simulink model "sldemo_hydcyl"  (Simulink 7.6)
settings: Solver=ode45  SolverMode=SingleTasking  StartTime=0  StopTime=0.1  RelTol=1e-4  AbsTol=1e-6
model workspace (MATLAB code in the model file):
  | % Load the initial conditions and initialization data
  | % Using the same MAT file as
  | % sldemo_hydcyl.mdl
  | % sldemo_hydcyl4.mdl
  | % sldemo_hydrod.mdl
  | 
  | load sldemo_hydcyl_data;
undefined symbols (not defined in the file or in its folder): C2, K, Qmax
libraries: hydlib x2
Description:
  | Single Hydraulic Cylinder Simulation
  | 
  | This demo uses Simulink(R) to model a hydraulic cylinder. You can apply these
  | concepts to applications where you need to model hydraulic behavior. See two
  | related demos that use the same basic components:
  | 
  | * four cylinder model: sldemo_hydcyl4.mdl
  | * two cylinder model with load constraints: sldemo_hydrod.mdl
settings Model: Creator=The MathWorks Inc.  CovMetricSettings=d  ExtModeTrigMode=oneshot  ExtModeArmWhenConnect=off  ExtModeAutoUpdateStatusClock=off  BufferReuse=off
settings DataIOCC: LimitDataPoints=off  SaveOutput=off  SaveTime=off  SignalLoggingName=sldemo_hydcyl_output
settings OptimizationCC: BlockReduction=off  BooleanDataType=off  ConditionallyExecuteInputs=off  InlineInvariantSignals=on  OptimizeBlockIOStorage=off  BufferReuse=off  ExpressionFolding=off  LocalBlockOutputs=off  InitFltsAndDblsToZero=on  BufferReusableBoundary=off
settings DebuggingCC: AlgebraicLoopMsg=none  SaveWithParameterizedLinksMsg=none  SignalResolutionControl=TryResolveAllWithWarning  SolverPrmCheckMsg=none  MultiTaskDSMMsg=warning  MultiTaskCondExecSysMsg=none  SigSpecEnsureSampleTimeMsg=none  IntegerOverflowMsg=none  BusObjectLabelMismatch=none
settings HardwareCC: TargetUnknown=on
settings RTWCC: IncludeERTFirstTime=on
settings GRTTargetCC: TargetFcnLib=ansi_tfl_tmw.mat

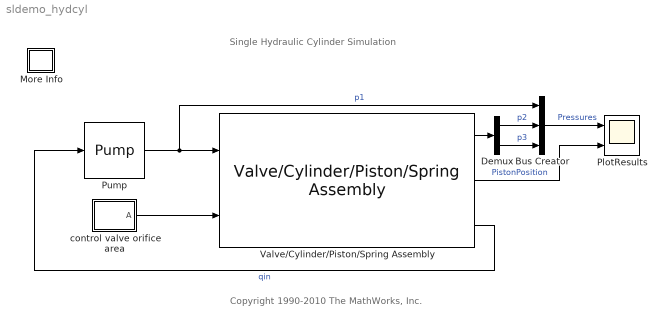
== system sldemo_hydcyl ==
  note: Single Hydraulic Cylinder Simulation
  note: Copyright 1990-2010 The MathWorks, Inc.
  Bus Creator : BusCreator  Inputs=3
  Demux : Demux  Outputs=2
  More Info : Subsystem
      settings: OpenFcn=showdemo(bdroot(gcs))
      mask Display: disp('?')
  PlotResults : Scope  NumInputPorts=2
      settings: TickLabels=on  TimeRange=0.1  YMin=0~0  YMax=2000000~0.04  DataFormat=Array
  Pump : hydlib/Pump  SystemSampleTime=-1  t="[0        .04     .04     .05    .05     .1]"  Qpump=Qmax*[1 1 0 0 1 1]  p10=Qmax/C2*2  C2=C2
  Valve/Cylinder/Piston/Spring Assembly : hydlib/Valve//Cylinder//Piston//Spring Assembly  SystemSampleTime=-1  K=K  C1=C1  Ac=Ac  Cd=Cd  rho=rho  V30=V30  beta=Beta  assemblyName=Spring
  control valve orifice area : Subsystem
      mask Type: Ramp
      mask Display: plot(0,0,100,100,[98,0],[96,0])
  wires:
  control valve orifice area/1(A) -> Valve/Cylinder/Piston/Spring Assembly/2
  Pump/1 -> Valve/Cylinder/Piston/Spring Assembly/1, Bus Creator/1  "p1"
  Valve/Cylinder/Piston/Spring Assembly/2 -> PlotResults/2  "PistonPosition"
  Valve/Cylinder/Piston/Spring Assembly/3 -> Pump/1  "qin"
  Valve/Cylinder/Piston/Spring Assembly/1 -> Demux/1
  Demux/1 -> Bus Creator/2  "p2"
  Demux/2 -> Bus Creator/3  "p3"
  Bus Creator/1 -> PlotResults/1  "Pressures"

== system sldemo_hydcyl/More Info ==

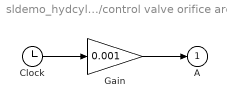
== system sldemo_hydcyl/control valve orifice area ==
  Clock : Clock
      settings: Decimation=10
  Gain : Gain  Gain=0.001  SaturateOnIntegerOverflow=on  OutDataTypeStr=Inherit: Same as input  ParamDataTypeStr=Inherit: Same as input
  A : Outport  InitialOutput=0
  wires:
  Gain/1 -> A/1
  Clock/1 -> Gain/1
